simulink model "netraSetuPipeline"  (R2026a)
settings: Solver=VariableStepAuto  StopTime=57600
PreLoadFcn:
  | buildFullEntityBus;
undefined symbols (not defined in the file or in its folder): m, n
settings Model: PacingRate=200  Creator=Tanuj  LastModifiedBy=Tanuj

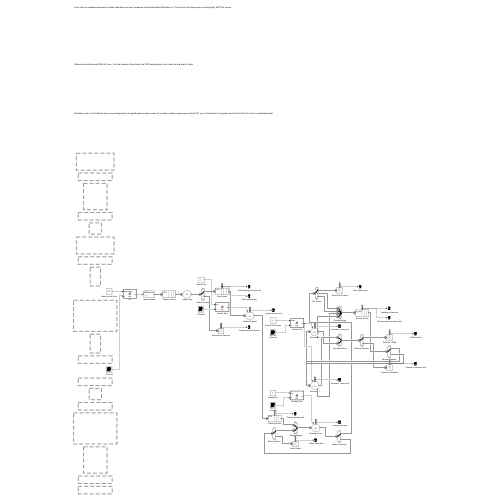
[thumbnail: Simulink's stored preview of the top-level diagram]
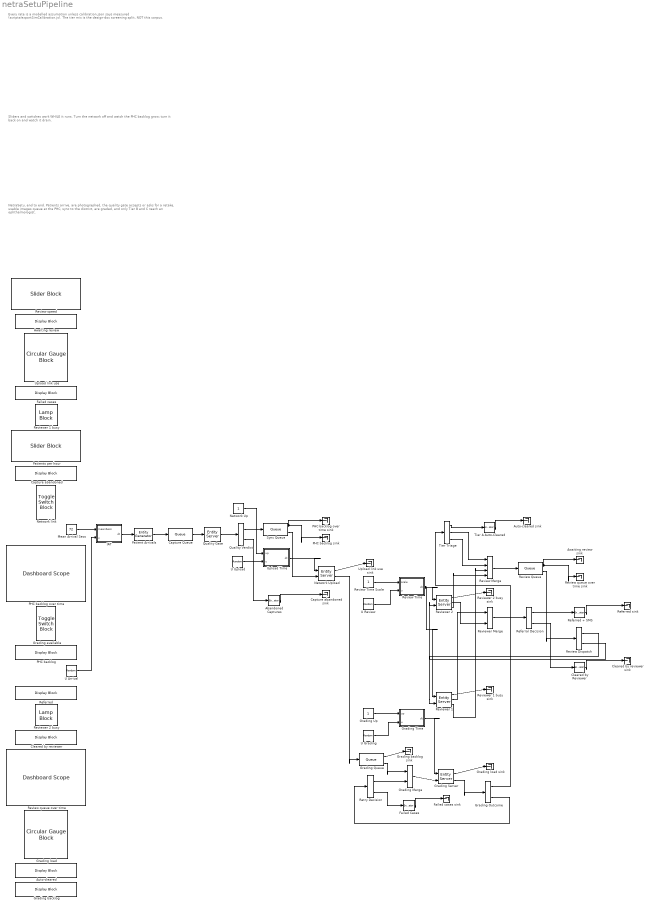
== system netraSetuPipeline ==
  note: NetraSetu, end to end. Patients arrive, are photographed, the quality gate accepts or asks for a retake, usable images queue at the PHC, sync to the district, are graded, and only Tier B and C reach an ophthalmologist.
  note: Sliders and switches work WHILE it runs. Turn the network off and watch the PHC backlog grow; turn it back on and watch it drain.
  note: Every rate is a modelled assumption unless calibration.json says measured (scripts/exportSimCalibration.js). The tier mix is the design-doc screening split, NOT this corpus.
  Abandoned Captures : EntityTerminator  InputPortMessageModes=m  NumberEntitiesArrived=on
      settings: OutputPortMap=o0
  Auto-cleared : DisplayBlock  LabelPosition=Hide  Transparency=1  GridColor=[0.502, 0.502, 0.502]
  Auto-cleared sink : Terminator
  Awaiting review : DisplayBlock  LabelPosition=Hide  Transparency=1  GridColor=[0.502, 0.502, 0.502]
  Awaiting review sink : Terminator
  Capture Queue : Queue  InputPortMessageModes=m  OutputPortMessageModes=m  Capacity=200
  Capture abandoned : DisplayBlock  LabelPosition=Hide  Transparency=1  GridColor=[0.502, 0.502, 0.502]
  Capture abandoned sink : Terminator
  Cleared by Reviewer : EntityTerminator  InputPortMessageModes=m  NumberEntitiesArrived=on
      settings: OutputPortMap=o0
  Cleared by reviewer : DisplayBlock  LabelPosition=Hide  Transparency=1  GridColor=[0.502, 0.502, 0.502]
  Cleared by reviewer sink : Terminator
  Failed Cases : EntityTerminator  InputPortMessageModes=m  NumberEntitiesArrived=on
      settings: OutputPortMap=o0
  Failed cases : DisplayBlock  LabelPosition=Hide  Transparency=1  GridColor=[0.502, 0.502, 0.502]
  Failed cases sink : Terminator
  Grading Merge : EntityInputSwitch  InputPortMessageModes=m,m  OutputPortMessageModes=m
  Grading Outcome : EntityOutputSwitch  InputPortMessageModes=m  OutputPortMessageModes=m,m  SwitchingCriterion=From attribute  SwitchAttributeName=failed
  Grading Queue : Queue  InputPortMessageModes=m  OutputPortMessageModes=n,m  Capacity=5000  NumberEntitiesInBlock=on
      settings: OutputPortMap=o1,o5
  Grading Server : EntityServer  InputPortMessageModes=n,m  OutputPortMessageModes=n,m  Capacity=2  ServiceTimeSource=Signal port  ServiceCompleteAction=|  Utilization=on
      | entity.attempts = entity.attempts + 1;
      | if rand() < 0.050000
      |   entity.failed = 2;
      | else
      |   entity.failed = 1;
      | end
      | if entity.attempts >= 3
      |   entity.route = 2;
      | else
      |   entity.route = 1;
      | end
      settings: InputPortMap=u0,u2  OutputPortMap=o5,o9
  Grading Time : MATLAB Function  TreatAsAtomicUnit=on
  Grading Up : Constant  SampleTime=1
  Grading available : ToggleSwitchBlock
  Grading backlog : DisplayBlock  LabelPosition=Hide  Transparency=1  GridColor=[0.502, 0.502, 0.502]
  Grading backlog sink : Terminator
  Grading load : CircularGaugeBlock  FontColor=[0.0, 0.0, 0.0]
  Grading load sink : Terminator
  IAT : MATLAB Function  TreatAsAtomicUnit=on
  Mean Arrival Secs : Constant  Value=72  SampleTime=1
  Network Up : Constant  SampleTime=1
  Network Upload : EntityServer  InputPortMessageModes=n,m  OutputPortMessageModes=n,m  Capacity=10  ServiceTimeSource=Signal port  Utilization=on
      settings: InputPortMap=u0,u2  OutputPortMap=o5,o9
  Network link : ToggleSwitchBlock
  PHC backlog : DisplayBlock  LabelPosition=Hide  Transparency=1  GridColor=[0.502, 0.502, 0.502]
  PHC backlog over time : DashboardScope  FontColor=[0.0, 0.0, 0.0]
  PHC backlog over time sink : Terminator
  PHC backlog sink : Terminator
  Patient Arrivals : EntityGenerator  OutputPortMessageModes=m  TimeSource=Signal port  GenerateAction=|  EntityType=Bus object  EntityTypeName=DRCaseFull
      | u = rand();
      | if u < 0.384057
      |   entity.prio = 1;
      | elseif u < 0.821605
      |   entity.prio = 2;
      | else
      |   entity.prio = 3;
      | end
      | entity.retakes = 0;
      | entity.attempts = 0;
      | entity.qc = 1;
      | entity.failed = 1;
      | entity.route = 1;
      | entity.refer = 2;
      settings: InputPortMap=u1
  Patients per hour : SliderBlock  ScaleMin=30  ScaleMax=600
  Quality Gate : EntityServer  InputPortMessageModes=m  OutputPortMessageModes=m  Capacity=10  ServiceTimeSource=MATLAB action  ServiceTimeAction=dt = 90 * (1 + entity.retakes);  EntryAction=|
      | n = 0;
      | ok = rand() < 0.925926;
      | while ~ok && n < 3
      |   n = n + 1;
      |   ok = rand() < 0.925926;
      | end
      | entity.retakes = n;
      | if ok
      |   entity.qc = 1;
      | else
      |   entity.qc = 2;
      | end
  Quality Verdict : EntityOutputSwitch  InputPortMessageModes=m  OutputPortMessageModes=m,m  SwitchingCriterion=From attribute  SwitchAttributeName=qc
  Referral Decision : EntityOutputSwitch  InputPortMessageModes=m  OutputPortMessageModes=m,m  SwitchingCriterion=From attribute  SwitchAttributeName=refer
  Referred : DisplayBlock  LabelPosition=Hide  Transparency=1  GridColor=[0.502, 0.502, 0.502]
  Referred + SMS : EntityTerminator  InputPortMessageModes=m  NumberEntitiesArrived=on
      settings: OutputPortMap=o0
  Referred sink : Terminator
  Retry Decision : EntityOutputSwitch  InputPortMessageModes=m  OutputPortMessageModes=m,m  SwitchingCriterion=From attribute  SwitchAttributeName=route
  Review Dispatch : EntityOutputSwitch  InputPortMessageModes=m  OutputPortMessageModes=m,m  SwitchAttributeName=Attribute1
  Review Merge : EntityInputSwitch  InputPortMessageModes=m,m,m,m  OutputPortMessageModes=m  NumberInputPorts=4
      settings: InputPortMap=u1,u2,u3,u4
  Review Queue : Queue  InputPortMessageModes=m  OutputPortMessageModes=n,m  Capacity=5000  QueueType=Priority  PrioritySource=prio  SortingDirection=Descending  NumberEntitiesInBlock=on
      settings: OutputPortMap=o1,o5
  Review Time : MATLAB Function  TreatAsAtomicUnit=on
  Review Time Scale : Constant  SampleTime=1
  Review queue over time : DashboardScope  FontColor=[0.0, 0.0, 0.0]
  Review queue over time sink : Terminator
  Review speed : SliderBlock  ScaleMin=0.25  ScaleMax=3
  Reviewer 1 : EntityServer  InputPortMessageModes=n,m  OutputPortMessageModes=n,m,m  Capacity=1  ServiceTimeSource=Signal port  ServiceCompleteAction=|  PermitPreemptionBasedOnAttribute=on  SortingAttributeName=prio  SortingDirection=Descending  WriteResidualTimeToAttribute=on  ResidualTimeAttributeName=residual  Utilization=on
      | if entity.prio >= 3
      |   entity.refer = 1;
      | elseif rand() < 0.300000
      |   entity.refer = 1;
      | else
      |   entity.refer = 2;
      | end
      settings: InputPortMap=u0,u2  OutputPortMap=o5,o9,o10
  Reviewer 1 busy : LampBlock  LabelPosition=Hide  DefaultColor=[192.0, 192.0, 192.0]
  Reviewer 1 busy sink : Terminator
  Reviewer 2 : EntityServer  InputPortMessageModes=n,m  OutputPortMessageModes=n,m,m  Capacity=1  ServiceTimeSource=Signal port  ServiceCompleteAction=|  PermitPreemptionBasedOnAttribute=on  SortingAttributeName=prio  SortingDirection=Descending  WriteResidualTimeToAttribute=on  ResidualTimeAttributeName=residual  Utilization=on
      | if entity.prio >= 3
      |   entity.refer = 1;
      | elseif rand() < 0.300000
      |   entity.refer = 1;
      | else
      |   entity.refer = 2;
      | end
      settings: InputPortMap=u0,u2  OutputPortMap=o5,o9,o10
  Reviewer 2 busy : LampBlock  LabelPosition=Hide  DefaultColor=[192.0, 192.0, 192.0]
  Reviewer 2 busy sink : Terminator
  Reviewer Merge : EntityInputSwitch  InputPortMessageModes=m,m  OutputPortMessageModes=m
  Sync Queue : Queue  InputPortMessageModes=m  OutputPortMessageModes=n,m  Capacity=5000  NumberEntitiesInBlock=on
      settings: OutputPortMap=o1,o5
  Tier A Auto-Cleared : EntityTerminator  InputPortMessageModes=m  NumberEntitiesArrived=on
      settings: OutputPortMap=o0
  Tier Triage : EntityOutputSwitch  InputPortMessageModes=m  OutputPortMessageModes=m,m,m  NumberOutputPorts=3  SwitchingCriterion=From attribute  SwitchAttributeName=prio
      settings: OutputPortMap=o0,o1,o2
  U Arrival : UniformRandomNumber  Minimum=0.0001  Seed=8148  SampleTime=1
  U Grading : UniformRandomNumber  Minimum=0.0001  Seed=1270  SampleTime=1
  U Review : UniformRandomNumber  Minimum=0.0001  Seed=9134  SampleTime=1
  U Upload : UniformRandomNumber  Minimum=0.0001  Seed=9058  SampleTime=1
  Upload Time : MATLAB Function  TreatAsAtomicUnit=on
  Upload link use : CircularGaugeBlock  FontColor=[0.0, 0.0, 0.0]
  Upload link use sink : Terminator
  wires:
  Mean Arrival Secs/1 -> IAT/1(meanSecs)
  U Review/1 -> Review Time/2(u)
  U Upload/1 -> Upload Time/2(u)
  Network Up/1 -> Upload Time/1(up)
  U Grading/1 -> Grading Time/2(u)
  Grading Up/1 -> Grading Time/1(up)
  U Arrival/1 -> IAT/2(u)
  Review Queue/2 -> Review Dispatch/1
  Reviewer 1/2 -> Reviewer Merge/1
  IAT/1(dt) -> Patient Arrivals/1
  Quality Verdict/1 -> Sync Queue/1
  Quality Gate/1 -> Quality Verdict/1
  Capture Queue/1 -> Quality Gate/1
  Patient Arrivals/1 -> Capture Queue/1
  Quality Verdict/2 -> Abandoned Captures/1
  Grading Server/2 -> Grading Outcome/1
  Grading Queue/2 -> Grading Merge/1
  Sync Queue/1 -> PHC backlog over time sink/1, PHC backlog sink/1
  Sync Queue/2 -> Network Upload/2
  Upload Time/1(dt) -> Network Upload/1
  Abandoned Captures/1 -> Capture abandoned sink/1
  Grading Outcome/1 -> Tier Triage/1
  Grading Merge/1 -> Grading Server/2
  Network Upload/1 -> Upload link use sink/1
  Network Upload/2 -> Grading Queue/1
  Review Time Scale/1 -> Review Time/1(scale)
  Retry Decision/1 -> Grading Merge/2
  Grading Queue/1 -> Grading backlog sink/1
  Review Dispatch/1 -> Reviewer 1/2
  Tier Triage/3 -> Review Merge/2
  Retry Decision/2 -> Failed Cases/1
  Review Time/1(dt) -> Reviewer 2/1, Reviewer 1/1
  Grading Time/1(dt) -> Grading Server/1
  Tier A Auto-Cleared/1 -> Auto-cleared sink/1
  Failed Cases/1 -> Failed cases sink/1
  Reviewer 1/1 -> Reviewer 1 busy sink/1
  Tier Triage/1 -> Tier A Auto-Cleared/1
  Review Merge/1 -> Review Queue/1
  Reviewer 1/3 -> Review Merge/3
  Tier Triage/2 -> Review Merge/1
  Referral Decision/1 -> Referred + SMS/1
  Reviewer 2/1 -> Reviewer 2 busy sink/1
  Reviewer 2/2 -> Reviewer Merge/2
  Referral Decision/2 -> Cleared by Reviewer/1
  Reviewer 2/3 -> Review Merge/4
  Grading Server/1 -> Grading load sink/1
  Reviewer Merge/1 -> Referral Decision/1
  Grading Outcome/2 -> Retry Decision/1
  Review Queue/1 -> Awaiting review sink/1, Review queue over time sink/1
  Referred + SMS/1 -> Referred sink/1
  Review Dispatch/2 -> Reviewer 2/2
  Cleared by Reviewer/1 -> Cleared by reviewer sink/1

== matlab function netraSetuPipeline/IAT ==
  data: meanSecs input; u input; dt output
function dt = fcn(meanSecs, u)
%#codegen
% inter-arrival time, exponential with a live mean.
uu = min(max(u, 1e-9), 1);
dt = -double(meanSecs) * log(uu);
dt = max(dt, 1e-3);

== matlab function netraSetuPipeline/Upload Time ==
  data: up input; u input; dt output
function dt = fcn(up, u)
%#codegen
% network upload time. up <= 0.5 means the stage is down.
uu = min(max(u, 1e-9), 1);
if up > 0.5
  dt = -29.6 * log(uu);
else
  dt = 1e6;
end
dt = max(dt, 1e-3);

== matlab function netraSetuPipeline/Grading Time ==
  data: up input; u input; dt output
function dt = fcn(up, u)
%#codegen
% grading time. up <= 0.5 means the stage is down.
uu = min(max(u, 1e-9), 1);
if up > 0.5
  dt = -39 * log(uu);
else
  dt = 1e6;
end
dt = max(dt, 1e-3);

== matlab function netraSetuPipeline/Review Time ==
  data: scale input; u input; dt output
function dt = fcn(scale, u)
%#codegen
% review service time, exponential, mean 30 s scaled live.
uu = min(max(u, 1e-9), 1);
dt = -(30 * double(scale)) * log(uu);
dt = max(dt, 1e-3);
